simulink model "ControllerModel"  (R2016a)
settings: Solver=VariableStepAuto  StartTime=0.0  StopTime=20  RelTol=1e-3
settings Model: Creator=lucas  LastModifiedBy=lucas

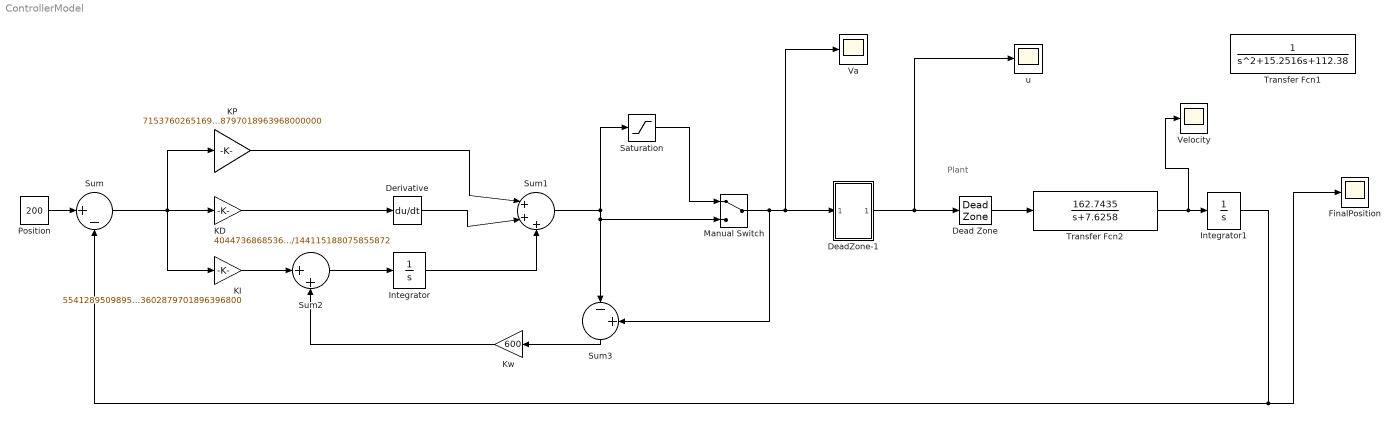
== system ControllerModel ==
  note: Plant
  Dead Zone : DeadZone  LowerValue=-0.02695  UpperValue=0.5449  ZeroCross=off  SaturateOnIntegerOverflow=on
  DeadZone-1 : Subsystem
  Derivative : Derivative
  FinalPosition : Scope
  Integrator : Integrator
  Integrator1 : Integrator
  KD : Gain  Gain=4044736868536971/144115188075855872
  KI : Gain  Gain=554128950989565027/3602879701896396800
  KP : Gain  Gain=7153760265169730591889/36028797018963968000000
  Kw : Gain  Gain=600
  Manual Switch : ManualSwitch
  Position : Constant  Value=200
  Saturation : Saturate  UpperLimit=6  LowerLimit=-6
  Sum : Sum  Inputs=|+-
  Sum1 : Sum  Inputs=|+++
  Sum2 : Sum  Inputs=|++
  Sum3 : Sum  Inputs=|-+
  Transfer Fcn1 : TransferFcn  Denominator=[1 15.2516 112.38]
  Transfer Fcn2 : TransferFcn  Numerator=[162.7435]  Denominator="[1  7.6258]"
  Va : Scope
  Velocity : Scope
  u : Scope
  wires:
  KP/1 -> Sum1/1
  Derivative/1 -> Sum1/2
  KD/1 -> Derivative/1
  Integrator/1 -> Sum1/3
  Sum2/1 -> Integrator/1
  KI/1 -> Sum2/1
  Sum/1 -> KI/1, KP/1, KD/1
  Sum1/1 -> Manual Switch/2, Sum3/1, Saturation/1
  Sum3/1 -> Kw/1
  Kw/1 -> Sum2/2
  Manual Switch/1 -> DeadZone-1/1(In1), Va/1, Sum3/2
  DeadZone-1/1(Out1) -> u/1, Dead Zone/1
  Integrator1/1 -> FinalPosition/1, Sum/2
  Transfer Fcn2/1 -> Velocity/1, Integrator1/1
  Dead Zone/1 -> Transfer Fcn2/1
  Position/1 -> Sum/1
  Saturation/1 -> Manual Switch/1

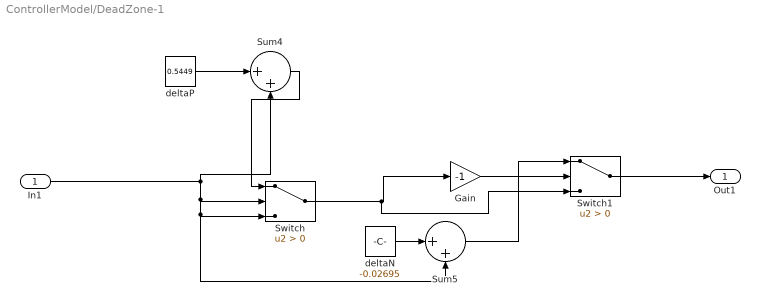
== system ControllerModel/DeadZone-1 ==
  In1 : Inport
  Gain : Gain  Gain=-1
  Sum4 : Sum  Inputs=|++
  Sum5 : Sum  Inputs=|++
  Switch : Switch  Criteria=u2 > Threshold
  Switch1 : Switch  Criteria=u2 > Threshold
  deltaN : Constant  Value=-0.02695
  deltaP : Constant  Value=0.5449
  Out1 : Outport
  wires:
  Sum4/1 -> Switch/1
  Switch/1 -> Switch1/3, Gain/1
  Sum5/1 -> Switch1/1
  Gain/1 -> Switch1/2
  deltaN/1 -> Sum5/1
  In1/1 -> Sum4/2, Switch/3, Sum5/2, Switch/2
  Switch1/1 -> Out1/1
  deltaP/1 -> Sum4/1
